simulink model "doc_moqpskdemod_sb"  (R2014a)
settings: Solver=FixedStepDiscrete  StartTime=0.0  StopTime=10.0  RelTol=1e-3
libraries: commdigbbndpm3 x2
settings Model: Creator=The MathWorks Inc.
settings DataIOCC: SignalLoggingSaveFormat=ModelDataLogs
settings OptimizationCC: BlockReduction=off  ExpressionDepthLimit=2147483647  EfficientMapNaN2IntZero=off
settings DebuggingCC: UnderspecifiedInitializationDetection=Classic  FcnCallInpInsideContextMsg=UseLocalSettings  StateNameClashWarn=warning  StrictBusMsg=Warning
settings GRTTargetCC: CombineOutputUpdateFcns=off  GRTInterface=on

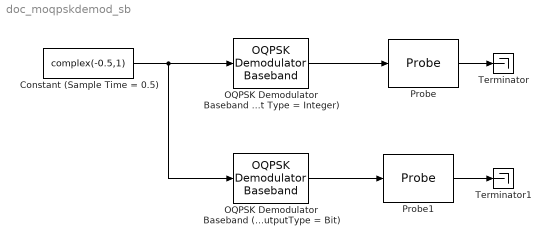
== system doc_moqpskdemod_sb ==
  Constant (Sample Time = 0.5) : Constant  Value=complex(-0.5,1)  VectorParams1D=off  SampleTime=0.5
  OQPSK Demodulator Baseband (Output Type = Integer) : commdigbbndpm3/OQPSK Demodulator Baseband  OutType=Integer  Ph=0  RateOptions=Allow multirate processing  outDtype1=Inherit via internal rule  outDtype2=double  derotateFactorWordLen=16  roundingMode=Floor  overflowMode=Wrap
  OQPSK Demodulator Baseband (OutputType = Bit) : commdigbbndpm3/OQPSK Demodulator Baseband  OutType=Bit  Ph=0  RateOptions=Allow multirate processing  outDtype1=double  outDtype2=double  derotateFactorWordLen=16  roundingMode=Floor  overflowMode=Wrap
  Probe : Probe  ProbeWidth=off  ProbeComplexSignal=off
  Probe1 : Probe  ProbeWidth=off  ProbeComplexSignal=off
  Terminator : Terminator
  Terminator1 : Terminator
  wires:
  Constant (Sample Time = 0.5)/1 -> OQPSK Demodulator Baseband (Output Type = Integer)/1, OQPSK Demodulator Baseband (OutputType = Bit)/1
  OQPSK Demodulator Baseband (Output Type = Integer)/1 -> Probe/1
  OQPSK Demodulator Baseband (OutputType = Bit)/1 -> Probe1/1
  Probe/1 -> Terminator/1
  Probe1/1 -> Terminator1/1
